simulink model "modelPartage2"  (Simulink 7.5)
settings: Solver=ode45  StartTime=0.0  StopTime=inf  RelTol=1e-3
settings Model: Creator=paris  LastModifiedBy=paris

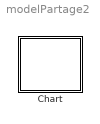
== system modelPartage2 ==
  Chart : Stateflow chart  TreatAsAtomicUnit=on

== stateflow chart Chart ==
  state MODEL ACTIVITE SITUEE [parallel]
    settings: executionOrder=1
    state Debut Situation
    state franchissement VAG
      state Approche
        Virage
      state Entree
        Virage
      state Debut Gestion
        Courbe
      state Fin Gestion
        Courbe
      state Sortie
        Virage
      MODEL.franchissement.Approche -> MODEL.franchissement.Entree : [ml.distPtA<=10]
      MODEL.franchissement.Entree -> MODEL.franchissement.Debut Gestion : [ml.distPtA==0]
      MODEL.franchissement.Debut Gestion -> MODEL.franchissement.Fin Gestion : [ml.distPtB==0]
      MODEL.franchissement.Fin Gestion -> MODEL.franchissement.Sortie : [ml.distPtC==0]
      (default) -> MODEL.franchissement.Approche : [ml.distPtA<=50]
    state gestion obstacle
      state Approche
        Obstacle
      state Depassement
        state Debut Dep
        state Fin Dep
      state Evitement
        state Fin Evit
        state Debut Evit
      (default) -> MODEL.gestion.Approche
      MODEL.gestion.Approche -> Depassement [order 1]
      MODEL.gestion.Approche -> Evitement [order 2]
    state cas témoin (sans SV)
    state Fin Situation
    state franchissement VAD
      state Entree
        Virage
      state Sortie
        Virage
      state Approche
        Virage
      state Fin Gestion
        Courbe
      state Debut Gestion
        Courbe
      MODEL.franchissement.Debut Gestion -> MODEL.franchissement.Fin Gestion : [ml.distPtB==0]
      MODEL.franchissement.Approche -> MODEL.franchissement.Entree : [ml.distPtA<=10]
      (default) -> MODEL.franchissement.Approche : [ml.distPtA<=50]
      MODEL.franchissement.Entree -> MODEL.franchissement.Debut Gestion : [ml.distPtA==0]
      MODEL.franchissement.Fin Gestion -> MODEL.franchissement.Sortie : [ml.distPtC==0]
    MODEL.franchissement.Sortie -> Fin Situation : [ml.type_infrastructure==62 + 3 secondes]
    franchissement VAD -> Fin Situation : [ml.type_infrastructure==62 + 3 secondes]
    Fin Dep -> Fin Situation : [ml.progression_SV==0]
    Fin Evit -> Fin Situation : [ml.progression_SV==0]
    Debut Situation -> cas témoin (sans SV) [order 4]
    (default) -> Debut Situation
    Debut Situation -> franchissement VAG [order 2] : [ml.type_infrastructure<=61]
    Debut Situation -> gestion obstacle [order 1] : [ml.etat_obstacle>0]
    Debut Situation -> franchissement VAD [order 3] : [ml.type_infrastructure>=63]
  state JUGEMENT ADEQUATION [parallel]
    settings: executionOrder=2
    state ? [parallel]
      settings: executionOrder=2
      state Sortie Voie Optimisation
      state Sortie Voie Defaut
    state ? [parallel]
      settings: executionOrder=1
      state Manoeuvres Tactiques
        Attendues
      state Actions Anormales
      state Manoeuvres Tactiques Anormales
      state Actions Attendues
  state DIAGNOSTIC SORTIE DE VOIE [parallel]
    settings: executionOrder=3
    state SORTIE DE VOIE (LEGITIMITE - CRITICITE)
      state LEGITIMITE [parallel]
        settings: executionOrder=2
        state Legitime
        state Illegitime
        state Potentielle
      state CRITICITE [parallel]
        settings: executionOrder=1
        state Criticite Faible
        state Criticite Moyenne
        state Criticite Forte
      state PROBABILITE OCCURENCE [parallel]
        settings: executionOrder=3
        state SV_Possible
        state SV_Imminente
        state SV_Probable
    state NON SORTIE DE VOIE
  state MANOEUVRE SORTIE DE VOIE [parallel]
    settings: executionOrder=4
    state SORTIE DE VOIE GAUCHE (CENTRE)
      state DANS VOIE
      state IMMINENTE
      state HORS DE VOIE
        state Recentration
        state Excentration
        MANOEUVRE.SORTIE.HORS.Excentration -> MANOEUVRE.SORTIE.HORS.Recentration : [ml.progression_SV==-1]
      (default) -> MANOEUVRE.SORTIE.IMMINENTE [order 1] : [ml.tlcCalcule<=1]
      MANOEUVRE.SORTIE.IMMINENTE -> MANOEUVRE.SORTIE.HORS.Excentration : [ml.progression_SV==1]
      MANOEUVRE.SORTIE.HORS.Recentration -> MANOEUVRE.SORTIE.DANS VOIE : [ml.etat_SV==0]
      (default) -> (junction 66) [order 2] : [ml.progression_SV==1]
    state SORTIE DE VOIE DROITE (ACCOTEMENT)
      state HORS DE VOIE
        state Recentration
        state Excentration
        MANOEUVRE.SORTIE.HORS.Excentration -> MANOEUVRE.SORTIE.HORS.Recentration : [ml.progression_SV==-1]
      state IMMINENTE
      state DANS VOIE
      MANOEUVRE.SORTIE.HORS.Recentration -> MANOEUVRE.SORTIE.DANS VOIE : [ml.etat_SV==0]
      (default) -> MANOEUVRE.SORTIE.IMMINENTE : [ml.tlcCalcule<=1]
      MANOEUVRE.SORTIE.IMMINENTE -> MANOEUVRE.SORTIE.HORS.Excentration : [ml.progression_SV==1]
    (default) -> (junction 64) [order 1] : [ml.lateralisation_SV==1]
    (default) -> (junction 65) [order 2] : [ml.lateralisation_SV==-1]
